simulink model "nmpc_sim"  (R2022a)
settings: Solver=ode4  StartTime=0.0  StopTime=30  FixedStep=0.0005  RelTol=1e-3
model workspace (MAT data in the model file):
  deg2rad = 0.0174532925199
  g2ms2 = 9.81
  kph2ms = 0.277777777778
  rad2deg = 57.2957795131
  rpm2rads = 0.10471975512
values from neighbouring files (symbols this model uses):
  N = 30    [plot_sim_results.m]
  Ts = T/N    (= 0.05)    [plot_sim_results.m]
undefined symbols (not defined in the file or in its folder): index_max, kappar, lbx_0, n_s, np, nu, nx, param_traj_0, phir, s_star_0, sr, u_s, ubx_0, V_star_0, veh, vr, wl, wr, x0, x_s, xr, yr
libraries: simulink x1
settings Model: Creator=Ting  LastModifiedBy=Ting
settings SolverCC: AlgebraicLoopSolver=TrustRegion
settings DebuggingCC: ArithmeticOperatorsInVariantConditions=warning
settings SFSimCC: CustomCodeUndefinedFunction=UseInterfaceOnly
settings CodeAppCC: StateflowObjectComments=on

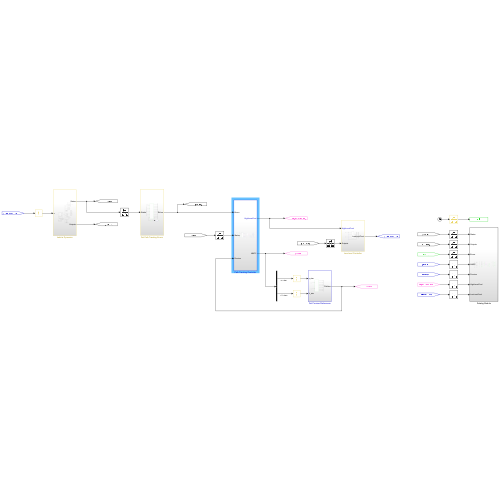
[thumbnail: Simulink's stored preview of the top-level diagram]
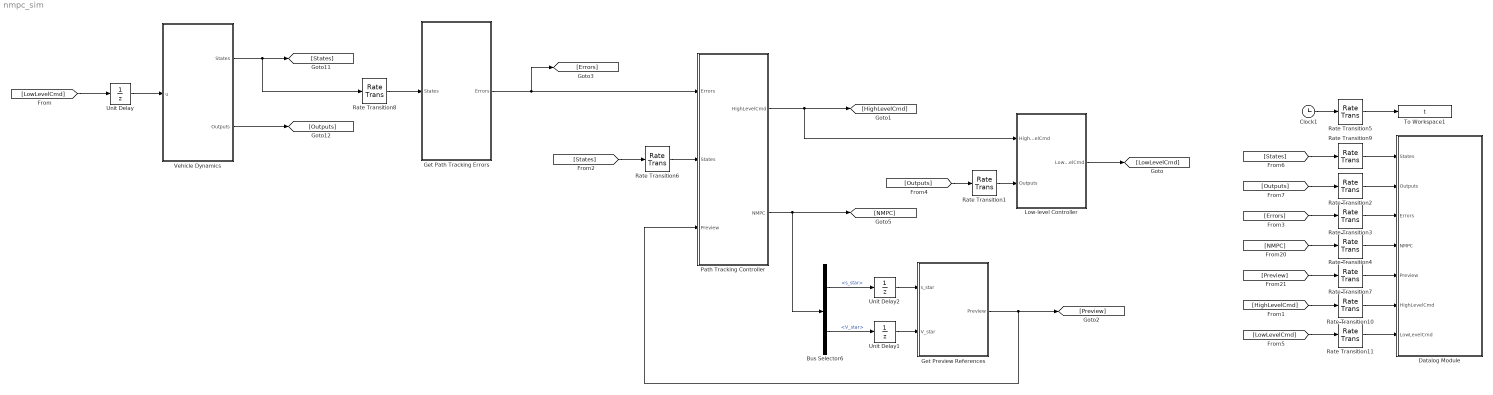
== system nmpc_sim ==
  Bus Selector6 : BusSelector  OutputSignals=s_star,V_star
  Clock1 : Clock
  Datalog Module : Subsystem
  "Get Path Tracking Errors " : Subsystem
  Get Preview References : Subsystem
  Low-level Controller : Subsystem
  Path Tracking Controller : Subsystem
  Rate Transition1 : RateTransition  OutPortSampleTime=Ts
  Rate Transition{2..5,7,9..11} (8 alike) : RateTransition  OutPortSampleTime=Ts_log
  Rate Transition6 : RateTransition  OutPortSampleTime=Ts
  Rate Transition8 : RateTransition  OutPortSampleTime=Ts
  To Workspace1 : ToWorkspace  VariableName=t  SampleTime=-1
      settings: Save2DSignal=2-D array (concatenate along first dimension)
  Unit Delay : UnitDelay  InitialCondition=zeros(7,1)  SampleTime=-1  HasFrameUpgradeWarning=on
  Unit Delay1 : UnitDelay  InitialCondition=V_star_0  SampleTime=-1  HasFrameUpgradeWarning=on
  Unit Delay2 : UnitDelay  InitialCondition=s_star_0  SampleTime=-1  HasFrameUpgradeWarning=on
  Vehicle Dynamics : Subsystem
  wires:
  Rate Transition5/1 -> To Workspace1/1
  Clock1/1 -> Rate Transition5/1
  [States] -> Rate Transition6/1
  Low-level Controller/1(LowLevelCmd) -> [LowLevelCmd]
  Path Tracking Controller/1(HighLevelCmd) -> Low-level Controller/1(HighLevelCmd), [HighLevelCmd]
  [Outputs] -> Rate Transition2/1
  [Outputs] -> Rate Transition1/1
  Unit Delay/1 -> Vehicle Dynamics/1(u)
  [Errors] -> Rate Transition3/1
  Get Preview References/1(Preview) -> Path Tracking Controller/3(Preview), [Preview]
  Rate Transition6/1 -> Path Tracking Controller/2(States)
  "Get Path Tracking Errors "/1(Errors) -> Path Tracking Controller/1(Errors), [Errors]
  Rate Transition8/1 -> "Get Path Tracking Errors "/1(States)
  Path Tracking Controller/2(NMPC) -> [NMPC], Bus Selector6/1
  Bus Selector6/2 -> Unit Delay1/1  "<V_star>"
  Bus Selector6/1 -> Unit Delay2/1  "<s_star>"
  [LowLevelCmd] -> Unit Delay/1
  Vehicle Dynamics/1(States) -> [States], Rate Transition8/1
  Vehicle Dynamics/2(Outputs) -> [Outputs]
  Unit Delay2/1 -> Get Preview References/1(s_star)
  Unit Delay1/1 -> Get Preview References/2(V_star)
  [States] -> Rate Transition9/1
  [HighLevelCmd] -> Rate Transition10/1
  [LowLevelCmd] -> Rate Transition11/1
  [NMPC] -> Rate Transition4/1
  [Preview] -> Rate Transition7/1
  Rate Transition9/1 -> Datalog Module/1(States)
  Rate Transition2/1 -> Datalog Module/2(Outputs)
  Rate Transition3/1 -> Datalog Module/3(Errors)
  Rate Transition4/1 -> Datalog Module/4(NMPC)
  Rate Transition7/1 -> Datalog Module/5(Preview)
  Rate Transition10/1 -> Datalog Module/6(HighLevelCmd)
  Rate Transition11/1 -> Datalog Module/7(LowLevelCmd)
  Rate Transition1/1 -> Low-level Controller/2(Outputs)

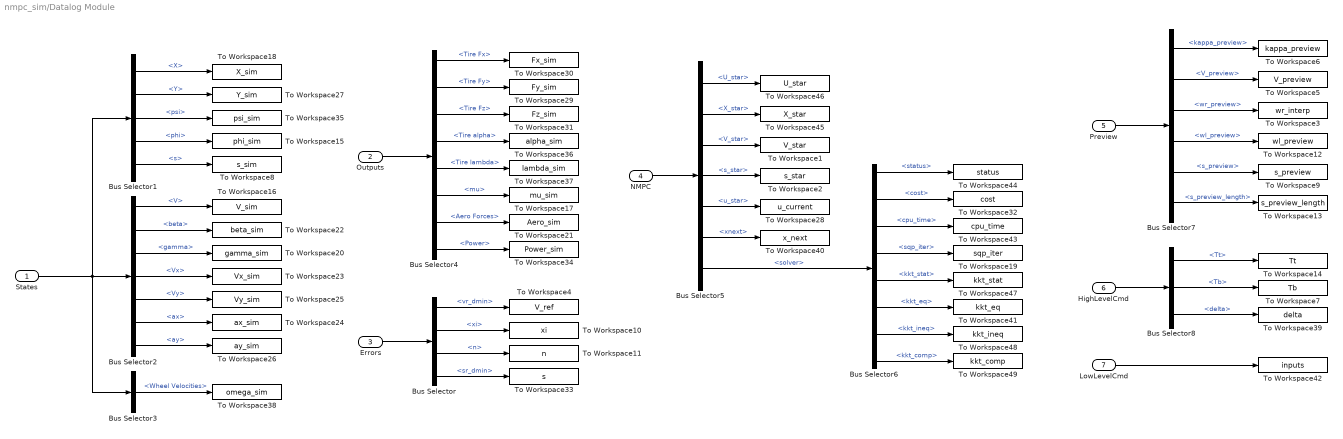
== system nmpc_sim/Datalog Module ==
  States : Inport
  Outputs : Inport  Port=2
  Errors : Inport  Port=3
  NMPC : Inport  Port=4
  Preview : Inport  Port=5
  HighLevelCmd : Inport  Port=6
  LowLevelCmd : Inport  Port=7
  Bus Selector : BusSelector  OutputSignals=vr_dmin,xi,n,sr_dmin
  Bus Selector1 : BusSelector  OutputSignals=Pose.X,Pose.Y,Pose.psi,Pose.phi,Pose.s
  Bus Selector2 : BusSelector  OutputSignals=Motion.V,Motion.beta,Motion.gamma,Motion.Vx,Motion.Vy,Motion.ax,Motion.ay
  Bus Selector3 : BusSelector  OutputSignals=Wheel Velocities
  Bus Selector4 : BusSelector  OutputSignals=Tire Fx,Tire Fy,Tire Fz,Tire alpha,Tire lambda,mu,Aero Forces,Power
  Bus Selector5 : BusSelector  OutputSignals=U_star,X_star,V_star,s_star,u_star,xnext,solver
  Bus Selector6 : BusSelector  OutputSignals=status,cost,cpu_time,sqp_iter,kkt_stat,kkt_eq,kkt_ineq,kkt_comp
  Bus Selector7 : BusSelector  OutputSignals=kappa_preview,V_preview,wr_preview,wl_preview,s_preview,s_preview_length
  Bus Selector8 : BusSelector  OutputSignals=Tt,Tb,delta
  To Workspace1 : ToWorkspace  VariableName=V_star  SampleTime=-1
  To Workspace10 : ToWorkspace  VariableName=xi  SampleTime=-1
  To Workspace11 : ToWorkspace  VariableName=n  SampleTime=-1
  To Workspace12 : ToWorkspace  VariableName=wl_preview  SampleTime=-1
  To Workspace13 : ToWorkspace  VariableName=s_preview_length  SampleTime=0.01
  To Workspace14 : ToWorkspace  VariableName=Tt  SampleTime=-1
      settings: Save2DSignal=2-D array (concatenate along first dimension)
  To Workspace15 : ToWorkspace  VariableName=phi_sim  SampleTime=-1
      settings: Save2DSignal=2-D array (concatenate along first dimension)
  To Workspace16 : ToWorkspace  VariableName=V_sim  SampleTime=-1
      settings: Save2DSignal=2-D array (concatenate along first dimension)
  To Workspace17 : ToWorkspace  VariableName=mu_sim  SampleTime=-1
  To Workspace18 : ToWorkspace  VariableName=X_sim  SampleTime=-1
      settings: Save2DSignal=2-D array (concatenate along first dimension)
  To Workspace19 : ToWorkspace  VariableName=sqp_iter  SampleTime=-1
      settings: Save2DSignal=2-D array (concatenate along first dimension)
  To Workspace2 : ToWorkspace  VariableName=s_star  SampleTime=-1
  To Workspace20 : ToWorkspace  VariableName=gamma_sim  SampleTime=-1
      settings: Save2DSignal=2-D array (concatenate along first dimension)
  To Workspace21 : ToWorkspace  VariableName=Aero_sim  SampleTime=-1
  To Workspace22 : ToWorkspace  VariableName=beta_sim  SampleTime=-1
      settings: Save2DSignal=2-D array (concatenate along first dimension)
  To Workspace23 : ToWorkspace  VariableName=Vx_sim  SampleTime=-1
      settings: Save2DSignal=2-D array (concatenate along first dimension)
  To Workspace24 : ToWorkspace  VariableName=ax_sim  SampleTime=-1
      settings: Save2DSignal=2-D array (concatenate along first dimension)
  To Workspace25 : ToWorkspace  VariableName=Vy_sim  SampleTime=-1
      settings: Save2DSignal=2-D array (concatenate along first dimension)
  To Workspace26 : ToWorkspace  VariableName=ay_sim  SampleTime=-1
      settings: Save2DSignal=2-D array (concatenate along first dimension)
  To Workspace27 : ToWorkspace  VariableName=Y_sim  SampleTime=-1
      settings: Save2DSignal=2-D array (concatenate along first dimension)
  To Workspace28 : ToWorkspace  VariableName=u_current  SampleTime=-1
      settings: Save2DSignal=2-D array (concatenate along first dimension)
  To Workspace29 : ToWorkspace  VariableName=Fy_sim  SampleTime=-1
  To Workspace3 : ToWorkspace  VariableName=wr_interp  SampleTime=-1
  To Workspace30 : ToWorkspace  VariableName=Fx_sim  SampleTime=-1
  To Workspace31 : ToWorkspace  VariableName=Fz_sim  SampleTime=-1
  To Workspace32 : ToWorkspace  VariableName=cost  SampleTime=-1
      settings: Save2DSignal=2-D array (concatenate along first dimension)
  To Workspace33 : ToWorkspace  VariableName=s  SampleTime=-1
  To Workspace34 : ToWorkspace  VariableName=Power_sim  SampleTime=-1
  To Workspace35 : ToWorkspace  VariableName=psi_sim  SampleTime=-1
      settings: Save2DSignal=2-D array (concatenate along first dimension)
  To Workspace36 : ToWorkspace  VariableName=alpha_sim  SampleTime=-1
  To Workspace37 : ToWorkspace  VariableName=lambda_sim  SampleTime=-1
  To Workspace38 : ToWorkspace  VariableName=omega_sim  SampleTime=-1
  To Workspace39 : ToWorkspace  VariableName=delta  SampleTime=-1
      settings: Save2DSignal=2-D array (concatenate along first dimension)
  To Workspace4 : ToWorkspace  VariableName=V_ref  SampleTime=-1
  To Workspace40 : ToWorkspace  VariableName=x_next  SampleTime=-1
      settings: Save2DSignal=2-D array (concatenate along first dimension)
  To Workspace41 : ToWorkspace  VariableName=kkt_eq  SampleTime=-1
      settings: Save2DSignal=2-D array (concatenate along first dimension)
  To Workspace42 : ToWorkspace  VariableName=inputs  SampleTime=-1
      settings: Save2DSignal=2-D array (concatenate along first dimension)
  To Workspace43 : ToWorkspace  VariableName=cpu_time  SampleTime=-1
      settings: Save2DSignal=2-D array (concatenate along first dimension)
  To Workspace44 : ToWorkspace  VariableName=status  SampleTime=-1
      settings: Save2DSignal=2-D array (concatenate along first dimension)
  To Workspace45 : ToWorkspace  VariableName=X_star  SampleTime=-1
  To Workspace46 : ToWorkspace  VariableName=U_star  SampleTime=-1
  To Workspace47 : ToWorkspace  VariableName=kkt_stat  SampleTime=-1
      settings: Save2DSignal=2-D array (concatenate along first dimension)
  To Workspace48 : ToWorkspace  VariableName=kkt_ineq  SampleTime=-1
      settings: Save2DSignal=2-D array (concatenate along first dimension)
  To Workspace49 : ToWorkspace  VariableName=kkt_comp  SampleTime=-1
      settings: Save2DSignal=2-D array (concatenate along first dimension)
  To Workspace5 : ToWorkspace  VariableName=V_preview  SampleTime=-1
  To Workspace6 : ToWorkspace  VariableName=kappa_preview  SampleTime=-1
  To Workspace7 : ToWorkspace  VariableName=Tb  SampleTime=-1
      settings: Save2DSignal=2-D array (concatenate along first dimension)
  To Workspace8 : ToWorkspace  VariableName=s_sim  SampleTime=-1
      settings: Save2DSignal=2-D array (concatenate along first dimension)
  To Workspace9 : ToWorkspace  VariableName=s_preview  SampleTime=-1
  wires:
  States/1 -> Bus Selector1/1, Bus Selector3/1, Bus Selector2/1
  Bus Selector2/5 -> To Workspace25/1  "<Vy>"
  Bus Selector1/2 -> To Workspace27/1  "<Y>"
  Bus Selector1/5 -> To Workspace8/1  "<s>"
  Bus Selector1/1 -> To Workspace18/1  "<X>"
  Bus Selector2/7 -> To Workspace26/1  "<ay>"
  Bus Selector1/3 -> To Workspace35/1  "<psi>"
  Bus Selector2/3 -> To Workspace20/1  "<gamma>"
  Bus Selector2/6 -> To Workspace24/1  "<ax>"
  Bus Selector1/4 -> To Workspace15/1  "<phi>"
  Bus Selector3/1 -> To Workspace38/1  "<Wheel Velocities>"
  Bus Selector2/2 -> To Workspace22/1  "<beta>"
  Bus Selector2/1 -> To Workspace16/1  "<V>"
  Bus Selector2/4 -> To Workspace23/1  "<Vx>"
  Bus Selector4/6 -> To Workspace17/1  "<mu>"
  Bus Selector4/3 -> To Workspace31/1  "<Tire Fz>"
  Bus Selector4/7 -> To Workspace21/1  "<Aero Forces>"
  Outputs/1 -> Bus Selector4/1
  Bus Selector4/5 -> To Workspace37/1  "<Tire lambda>"
  Bus Selector4/1 -> To Workspace30/1  "<Tire Fx>"
  Bus Selector4/4 -> To Workspace36/1  "<Tire alpha>"
  Bus Selector4/2 -> To Workspace29/1  "<Tire Fy>"
  Bus Selector4/8 -> To Workspace34/1  "<Power>"
  Bus Selector/2 -> To Workspace10/1  "<xi>"
  Bus Selector/4 -> To Workspace33/1  "<sr_dmin>"
  Bus Selector/1 -> To Workspace4/1  "<vr_dmin>"
  Bus Selector/3 -> To Workspace11/1  "<n>"
  Errors/1 -> Bus Selector/1
  NMPC/1 -> Bus Selector5/1
  Bus Selector5/1 -> To Workspace46/1  "<U_star>"
  Bus Selector5/2 -> To Workspace45/1  "<X_star>"
  Bus Selector5/3 -> To Workspace1/1  "<V_star>"
  Bus Selector5/4 -> To Workspace2/1  "<s_star>"
  Bus Selector5/5 -> To Workspace28/1  "<u_star>"
  Bus Selector5/6 -> To Workspace40/1  "<xnext>"
  Bus Selector5/7 -> Bus Selector6/1  "<solver>"
  Bus Selector6/1 -> To Workspace44/1  "<status>"
  Bus Selector6/2 -> To Workspace32/1  "<cost>"
  Bus Selector6/3 -> To Workspace43/1  "<cpu_time>"
  Bus Selector6/4 -> To Workspace19/1  "<sqp_iter>"
  Bus Selector6/5 -> To Workspace47/1  "<kkt_stat>"
  Bus Selector6/6 -> To Workspace41/1  "<kkt_eq>"
  Bus Selector6/7 -> To Workspace48/1  "<kkt_ineq>"
  Bus Selector6/8 -> To Workspace49/1  "<kkt_comp>"
  Preview/1 -> Bus Selector7/1
  Bus Selector7/1 -> To Workspace6/1  "<kappa_preview>"
  Bus Selector7/2 -> To Workspace5/1  "<V_preview>"
  Bus Selector7/3 -> To Workspace3/1  "<wr_preview>"
  Bus Selector7/4 -> To Workspace12/1  "<wl_preview>"
  Bus Selector7/5 -> To Workspace9/1  "<s_preview>"
  Bus Selector7/6 -> To Workspace13/1  "<s_preview_length>"
  Bus Selector8/3 -> To Workspace39/1  "<delta>"
  Bus Selector8/1 -> To Workspace14/1  "<Tt>"
  Bus Selector8/2 -> To Workspace7/1  "<Tb>"
  HighLevelCmd/1 -> Bus Selector8/1
  LowLevelCmd/1 -> To Workspace42/1

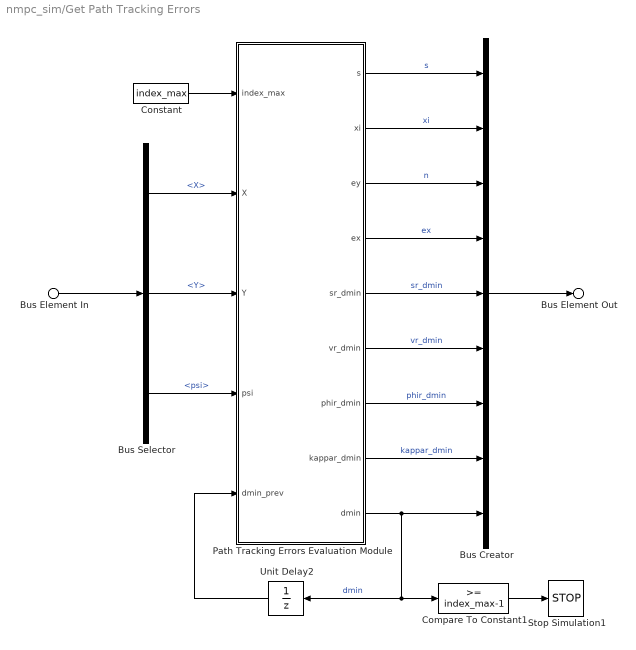
== system nmpc_sim/Get Path Tracking Errors  ==
  Bus Element In : Inport  PortName=States
  Bus Creator : BusCreator  Inputs=9
  Bus Selector : BusSelector  OutputSignals=Pose.X,Pose.Y,Pose.psi
  Compare To Constant1 : simulink/Logic and Bit Operations/Compare To Constant  relop=>=  const=index_max-1  OutDataTypeStr=boolean
  Constant : Constant  Value=index_max
  Path Tracking Errors Evaluation Module : MATLAB Function  TreatAsAtomicUnit=on
  Stop Simulation1 : Stop
  Unit Delay2 : UnitDelay  InitialCondition=1  SampleTime=-1  HasFrameUpgradeWarning=on
  Bus Element Out : Outport  PortName=Errors
  wires:
  Constant/1 -> Path Tracking Errors Evaluation Module/1(index_max)
  Bus Selector/1 -> Path Tracking Errors Evaluation Module/2(X)  "<X>"
  Bus Selector/2 -> Path Tracking Errors Evaluation Module/3(Y)  "<Y>"
  Bus Selector/3 -> Path Tracking Errors Evaluation Module/4(psi)  "<psi>"
  Path Tracking Errors Evaluation Module/9(dmin) -> Bus Creator/9, Unit Delay2/1, Compare To Constant1/1  "dmin"
  Unit Delay2/1 -> Path Tracking Errors Evaluation Module/5(dmin_prev)
  Path Tracking Errors Evaluation Module/2(xi) -> Bus Creator/2  "xi"
  Path Tracking Errors Evaluation Module/3(ey) -> Bus Creator/3  "n"
  Path Tracking Errors Evaluation Module/4(ex) -> Bus Creator/4  "ex"
  Path Tracking Errors Evaluation Module/5(sr_dmin) -> Bus Creator/5  "sr_dmin"
  Path Tracking Errors Evaluation Module/6(vr_dmin) -> Bus Creator/6  "vr_dmin"
  Path Tracking Errors Evaluation Module/7(phir_dmin) -> Bus Creator/7  "phir_dmin"
  Path Tracking Errors Evaluation Module/8(kappar_dmin) -> Bus Creator/8  "kappar_dmin"
  Bus Element In/1 -> Bus Selector/1
  Bus Creator/1 -> Bus Element Out/1
  Compare To Constant1/1 -> Stop Simulation1/1
  Path Tracking Errors Evaluation Module/1(s) -> Bus Creator/1  "s"

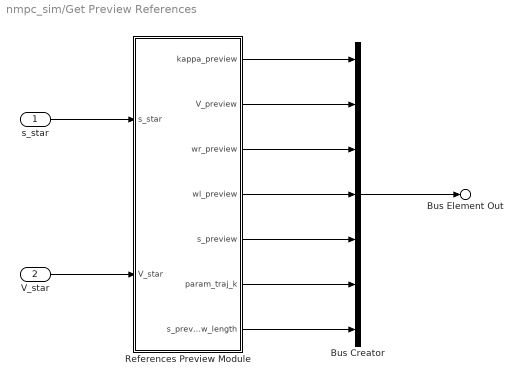
== system nmpc_sim/Get Preview References ==
  s_star : Inport
  V_star : Inport  Port=2
  Bus Creator : BusCreator  Inputs=7
  References Preview Module : MATLAB Function  TreatAsAtomicUnit=on
  Bus Element Out : Outport  PortName=Preview
  wires:
  s_star/1 -> References Preview Module/1(s_star)
  V_star/1 -> References Preview Module/2(V_star)
  References Preview Module/1(kappa_preview) -> Bus Creator/1
  References Preview Module/2(V_preview) -> Bus Creator/2
  References Preview Module/3(wr_preview) -> Bus Creator/3
  References Preview Module/4(wl_preview) -> Bus Creator/4
  References Preview Module/7(s_preview_length) -> Bus Creator/7
  References Preview Module/5(s_preview) -> Bus Creator/5
  References Preview Module/6(param_traj_k) -> Bus Creator/6
  Bus Creator/1 -> Bus Element Out/1

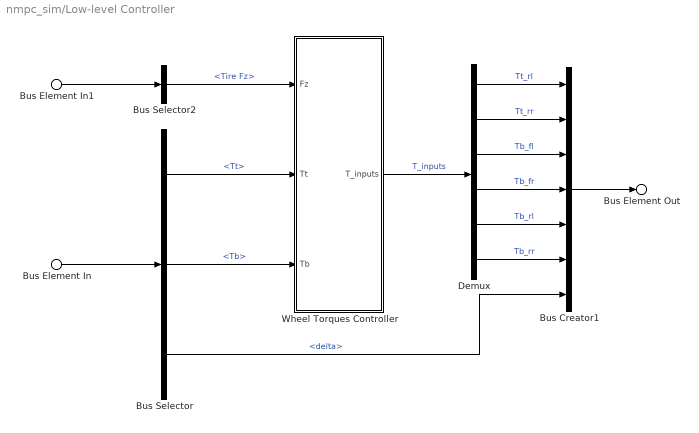
== system nmpc_sim/Low-level Controller ==
  Bus Element In : Inport  PortName=HighLevelCmd
  Bus Element In1 : Inport  Port=2  PortName=Outputs
  Bus Creator1 : BusCreator  Inputs=7
  Bus Selector : BusSelector  OutputSignals=Tt,Tb,delta
  Bus Selector2 : BusSelector  OutputSignals=Tire Fz
  Demux : Demux  Outputs=6
  "Wheel Torques Controller " : MATLAB Function  TreatAsAtomicUnit=on
  Bus Element Out : Outport  PortName=LowLevelCmd
  wires:
  Bus Element In/1 -> Bus Selector/1
  Bus Selector/1 -> "Wheel Torques Controller "/2(Tt)  "<Tt>"
  Bus Selector/2 -> "Wheel Torques Controller "/3(Tb)  "<Tb>"
  "Wheel Torques Controller "/1(T_inputs) -> Demux/1  "T_inputs"
  Bus Element In1/1 -> Bus Selector2/1
  Bus Selector2/1 -> "Wheel Torques Controller "/1(Fz)  "<Tire Fz>"
  Demux/1 -> Bus Creator1/1  "Tt_rl"
  Demux/2 -> Bus Creator1/2  "Tt_rr"
  Demux/3 -> Bus Creator1/3  "Tb_fl"
  Demux/4 -> Bus Creator1/4  "Tb_fr"
  Bus Creator1/1 -> Bus Element Out/1
  Demux/5 -> Bus Creator1/5  "Tb_rl"
  Demux/6 -> Bus Creator1/6  "Tb_rr"
  Bus Selector/3 -> Bus Creator1/7  "<delta>"

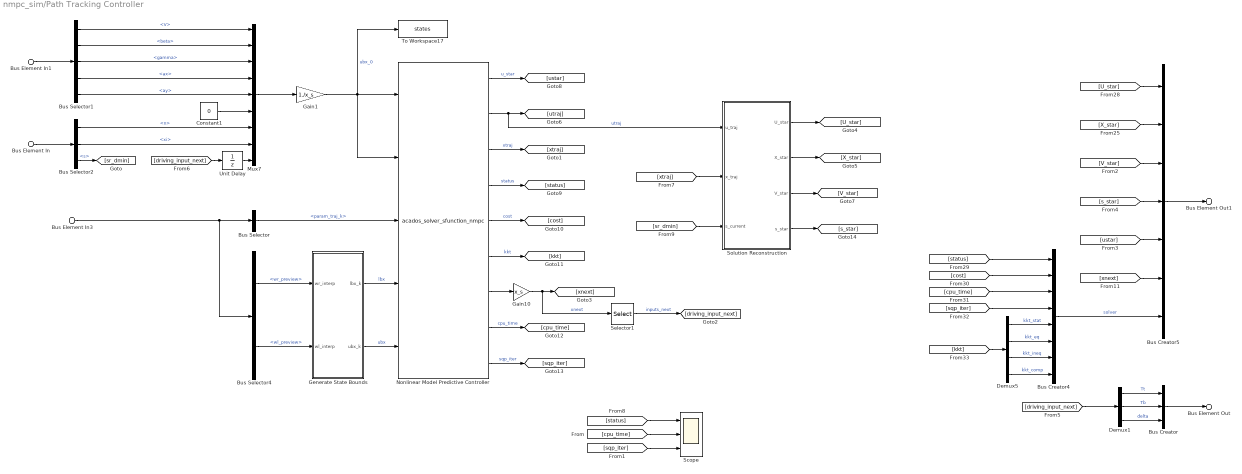
== system nmpc_sim/Path Tracking Controller ==
  Bus Element In : Inport  PortName=Errors
  Bus Element In1 : Inport  Port=2  PortName=States
  Bus Element In3 : Inport  Port=3  PortName=Preview
  Bus Creator : BusCreator  Inputs=3
  Bus Creator4 : BusCreator  Inputs=8
  Bus Creator5 : BusCreator  Inputs=7
  Bus Selector : BusSelector  OutputSignals=param_traj_k
  Bus Selector1 : BusSelector  OutputSignals=Motion.V,Motion.beta,Motion.gamma,Motion.ax,Motion.ay
  Bus Selector2 : BusSelector  OutputSignals=n,xi,s
  Bus Selector4 : BusSelector  OutputSignals=wr_preview,wl_preview
  Constant1 : Constant  Value=0
  Demux1 : Demux  Outputs=3
  Demux5 : Demux
  Gain1 : Gain  Gain=1./x_s
  Gain10 : Gain  Gain=x_s
  Generate State Bounds : MATLAB Function  TreatAsAtomicUnit=on
  Mux7 : Mux  Inputs=[1 1 1 1 1 1 1 1 3]
  Nonlinear Model Predictive Controller : S-Function  FunctionName=acados_solver_sfunction_nmpc  SFunctionDeploymentMode=off  EnableBusSupport=off
      mask Display:
      | global sfun_input_names sfun_output_names
      | for i = 1:length(sfun_input_names)
      | 	port_label('input', i, sfun_input_names{i})
      | end
      | for i = 1:length(sfun_output_names)
      | 	port_label('output', i, sfun_output_names{i})
      | end
  Scope : Scope  NumInputPorts=3
  Selector1 : Selector  InputPortWidth=11  IndexOptions=Index vector (dialog)  Indices=[9 10 11]  OutputSizes=1
  Solution Reconstruction : MATLAB Function  TreatAsAtomicUnit=on
  To Workspace17 : ToWorkspace  VariableName=states  SampleTime=-1
      settings: Save2DSignal=2-D array (concatenate along first dimension)
  Unit Delay : UnitDelay  InitialCondition=[0 0 0]'  SampleTime=-1  HasFrameUpgradeWarning=on
  Bus Element Out : Outport  PortName=HighLevelCmd
  Bus Element Out1 : Outport  Port=2  PortName=NMPC
  wires:
  Nonlinear Model Predictive Controller/1 -> [ustar]  "u_star"
  Bus Selector1/2 -> Mux7/2  "<beta>"
  Bus Selector2/2 -> Mux7/8  "<xi>"
  Nonlinear Model Predictive Controller/9 -> [sqp_iter]  "sqp_iter"
  Gain1/1 -> Nonlinear Model Predictive Controller/1, Nonlinear Model Predictive Controller/2, To Workspace17/1  "ubx_0"
  Nonlinear Model Predictive Controller/8 -> [cpu_time]  "cpu_time"
  Bus Selector2/1 -> Mux7/7  "<n>"
  Mux7/1 -> Gain1/1
  Bus Selector1/1 -> Mux7/1  "<V>"
  Nonlinear Model Predictive Controller/7 -> Gain10/1
  Nonlinear Model Predictive Controller/2 -> Solution Reconstruction/1(u_traj), [utraj]  "utraj"
  Nonlinear Model Predictive Controller/3 -> [xtraj]  "xtraj"
  Nonlinear Model Predictive Controller/4 -> [status]  "status"
  Generate State Bounds/1(lbx_k) -> Nonlinear Model Predictive Controller/4  "lbx"
  Generate State Bounds/2(ubx_k) -> Nonlinear Model Predictive Controller/5  "ubx"
  Bus Element In1/1 -> Bus Selector1/1
  Bus Element In/1 -> Bus Selector2/1
  Unit Delay/1 -> Mux7/9
  [driving_input_next] -> Unit Delay/1
  Bus Selector1/3 -> Mux7/3  "<gamma>"
  Bus Selector1/4 -> Mux7/4  "<ax>"
  [xtraj] -> Solution Reconstruction/2(x_traj)
  Solution Reconstruction/3(V_star) -> [V_star]
  Solution Reconstruction/4(s_star) -> [s_star]
  Bus Selector1/5 -> Mux7/5  "<ay>"
  Bus Element In3/1 -> Bus Selector/1, Bus Selector4/1
  Bus Selector/1 -> Nonlinear Model Predictive Controller/3  "<param_traj_k>"
  Bus Selector4/1 -> Generate State Bounds/1(wr_interp)  "<wr_preview>"
  Bus Selector4/2 -> Generate State Bounds/2(wl_interp)  "<wl_preview>"
  Solution Reconstruction/1(U_star) -> [U_star]
  Solution Reconstruction/2(X_star) -> [X_star]
  Nonlinear Model Predictive Controller/6 -> [kkt]  "kkt"
  Nonlinear Model Predictive Controller/5 -> [cost]  "cost"
  Demux5/4 -> Bus Creator4/8  "kkt_comp"
  Demux5/3 -> Bus Creator4/7  "kkt_ineq"
  Demux5/1 -> Bus Creator4/5  "kkt_stat"
  Demux5/2 -> Bus Creator4/6  "kkt_eq"
  Gain10/1 -> Selector1/1, [xnext]  "xnext"
  [ustar] -> Bus Creator5/5
  [U_star] -> Bus Creator5/1
  [X_star] -> Bus Creator5/2
  [xnext] -> Bus Creator5/6
  [status] -> Bus Creator4/1
  [cost] -> Bus Creator4/2
  [kkt] -> Demux5/1
  [cpu_time] -> Bus Creator4/3
  [sqp_iter] -> Bus Creator4/4
  Bus Creator4/1 -> Bus Creator5/7  "solver"
  Bus Creator5/1 -> Bus Element Out1/1
  [V_star] -> Bus Creator5/3
  [s_star] -> Bus Creator5/4
  Selector1/1 -> [driving_input_next]  "inputs_next"
  Demux1/2 -> Bus Creator/2  "Tb"
  Bus Creator/1 -> Bus Element Out/1
  Demux1/3 -> Bus Creator/3  "delta"
  Demux1/1 -> Bus Creator/1  "Tt"
  [driving_input_next] -> Demux1/1
  [cpu_time] -> Scope/2
  [sqp_iter] -> Scope/3
  Constant1/1 -> Mux7/6
  [sr_dmin] -> Solution Reconstruction/3(s_current)
  Bus Selector2/3 -> [sr_dmin]  "<s>"
  [status] -> Scope/1

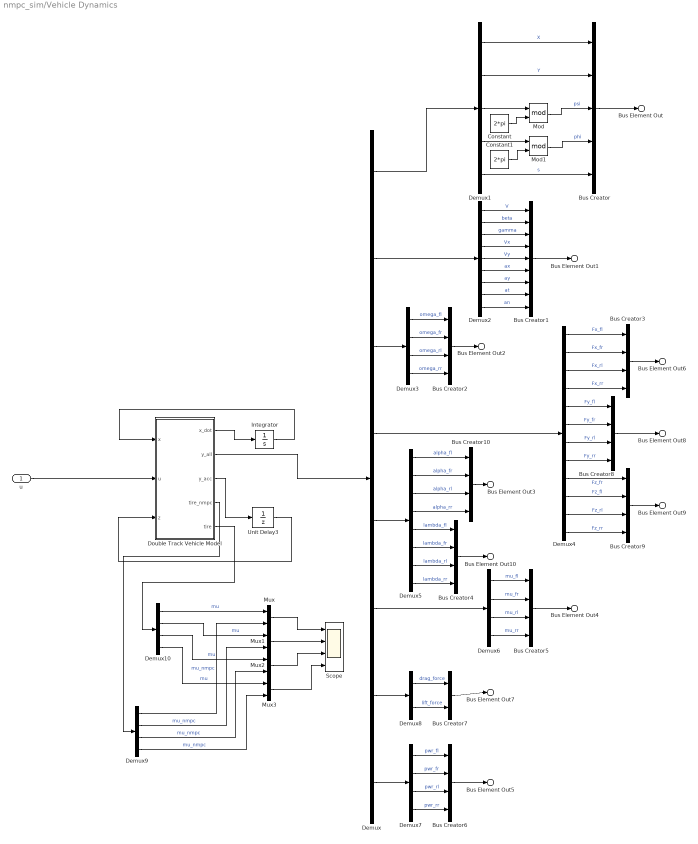
== system nmpc_sim/Vehicle Dynamics ==
  u : Inport
  Bus Creator : BusCreator  Inputs=5
  Bus Creator1 : BusCreator  Inputs=9
  Bus Creator{2..6,8..10} (8 alike) : BusCreator  Inputs=4
  Bus Creator7 : BusCreator  Inputs=2
  Constant : Constant  Value=2*pi
  Constant1 : Constant  Value=2*pi
  Demux : Demux  Outputs=[5 9 4 12 8 4 2 4]
  Demux1 : Demux  Outputs=5
  Demux{3,6..7,9..10} (5 alike) : Demux
  Demux2 : Demux  Outputs=9
  Demux4 : Demux  Outputs=12
  Demux5 : Demux  Outputs=8
  Demux8 : Demux  Outputs=2
  Double Track Vehicle Model : MATLAB Function  TreatAsAtomicUnit=on
  Integrator : Integrator  InitialCondition=x0
  Mod : Math  Operator=mod  SignedPower=on
  Mod1 : Math  Operator=mod  SignedPower=on
  Mux{,1..3} (4 alike) : Mux  Inputs=2
  Scope : Scope  NumInputPorts=4
  Unit Delay3 : UnitDelay  InitialCondition=[0; 0];  SampleTime=-1  HasFrameUpgradeWarning=on
  Bus Element Out : Outport  PortName=States  Element=Pose
  Bus Element Out2 : Outport  PortName=States  Element=Wheel Velocities
  Bus Element Out1 : Outport  PortName=States  Element=Motion
  Bus Element Out3 : Outport  Port=2  PortName=Outputs  Element=Tire alpha
  Bus Element Out4 : Outport  Port=2  PortName=Outputs  Element=mu
  Bus Element Out5 : Outport  Port=2  PortName=Outputs  Element=Power
  Bus Element Out7 : Outport  Port=2  PortName=Outputs  Element=Aero Forces
  Bus Element Out8 : Outport  Port=2  PortName=Outputs  Element=Tire Fy
  Bus Element Out6 : Outport  Port=2  PortName=Outputs  Element=Tire Fx
  Bus Element Out9 : Outport  Port=2  PortName=Outputs  Element=Tire Fz
  Bus Element Out10 : Outport  Port=2  PortName=Outputs  Element=Tire lambda
  wires:
  Double Track Vehicle Model/3(y_acc) -> Unit Delay3/1
  Unit Delay3/1 -> Double Track Vehicle Model/3(z)
  Double Track Vehicle Model/1(x_dot) -> Integrator/1
  Double Track Vehicle Model/2(y_all) -> Demux/1
  u/1 -> Double Track Vehicle Model/2(u)
  Integrator/1 -> Double Track Vehicle Model/1(x)
  Demux1/2 -> Bus Creator/2  "Y"
  Demux1/1 -> Bus Creator/1  "X"
  Demux1/3 -> Mod/1
  Demux1/4 -> Mod1/1
  Bus Creator/1 -> Bus Element Out/1
  Demux/2 -> Demux2/1
  Demux2/1 -> Bus Creator1/1  "V"
  Demux2/2 -> Bus Creator1/2  "beta"
  Demux2/3 -> Bus Creator1/3  "gamma"
  Demux2/4 -> Bus Creator1/4  "Vx"
  Demux2/5 -> Bus Creator1/5  "Vy"
  Demux2/6 -> Bus Creator1/6  "ax"
  Demux2/7 -> Bus Creator1/7  "ay"
  Bus Creator2/1 -> Bus Element Out2/1
  Demux3/4 -> Bus Creator2/4  "omega_rr"
  Demux3/3 -> Bus Creator2/3  "omega_rl"
  Demux3/1 -> Bus Creator2/1  "omega_fl"
  Demux3/2 -> Bus Creator2/2  "omega_fr"
  Demux/3 -> Demux3/1
  Demux/4 -> Demux4/1
  Demux4/1 -> Bus Creator3/1  "Fx_fl"
  Demux4/2 -> Bus Creator3/2  "Fx_fr"
  Demux4/3 -> Bus Creator3/3  "Fx_rl"
  Demux4/4 -> Bus Creator3/4  "Fx_rr"
  Demux4/5 -> Bus Creator8/1  "Fy_fl"
  Demux4/6 -> Bus Creator8/2  "Fy_fr"
  Demux4/7 -> Bus Creator8/3  "Fy_rl"
  Demux4/8 -> Bus Creator8/4  "Fy_rr"
  Demux4/9 -> Bus Creator9/1  "Fz_fr"
  Demux4/10 -> Bus Creator9/2  "Fz_fl"
  Demux4/11 -> Bus Creator9/3  "Fz_rl"
  Demux4/12 -> Bus Creator9/4  "Fz_rr"
  Bus Creator3/1 -> Bus Element Out6/1
  Bus Creator1/1 -> Bus Element Out1/1
  Demux/5 -> Demux5/1
  Demux5/1 -> Bus Creator10/1  "alpha_fl"
  Demux5/2 -> Bus Creator10/2  "alpha_fr"
  Demux5/3 -> Bus Creator10/3  "alpha_rl"
  Demux5/4 -> Bus Creator10/4  "alpha_rr"
  Demux5/5 -> Bus Creator4/1  "lambda_fl"
  Demux5/6 -> Bus Creator4/2  "lambda_fr"
  Demux5/7 -> Bus Creator4/3  "lambda_rl"
  Demux5/8 -> Bus Creator4/4  "lambda_rr"
  Bus Creator10/1 -> Bus Element Out3/1
  Demux/6 -> Demux6/1
  Demux6/2 -> Bus Creator5/2  "mu_fr"
  Demux6/3 -> Bus Creator5/3  "mu_rl"
  Demux6/4 -> Bus Creator5/4  "mu_rr"
  Bus Creator5/1 -> Bus Element Out4/1
  Demux6/1 -> Bus Creator5/1  "mu_fl"
  Bus Creator6/1 -> Bus Element Out5/1
  Demux7/4 -> Bus Creator6/4  "pwr_rr"
  Demux7/3 -> Bus Creator6/3  "pwr_rl"
  Demux7/2 -> Bus Creator6/2  "pwr_fr"
  Demux/8 -> Demux7/1
  Demux7/1 -> Bus Creator6/1  "pwr_fl"
  Demux/7 -> Demux8/1
  Demux8/1 -> Bus Creator7/1  "drag_force"
  Demux8/2 -> Bus Creator7/2  "lift_force"
  Bus Creator7/1 -> Bus Element Out7/1
  Demux1/5 -> Bus Creator/5  "s"
  Bus Creator8/1 -> Bus Element Out8/1
  Bus Creator9/1 -> Bus Element Out9/1
  Bus Creator4/1 -> Bus Element Out10/1
  Mod/1 -> Bus Creator/3  "psi"
  Constant/1 -> Mod/2
  Mod1/1 -> Bus Creator/4  "phi"
  Constant1/1 -> Mod1/2
  Demux/1 -> Demux1/1
  Double Track Vehicle Model/4(tire_nmpc) -> Demux9/1
  Demux9/1 -> Mux/2  "mu_nmpc"
  Demux9/2 -> Mux1/2  "mu_nmpc"
  Demux9/3 -> Mux2/2  "mu_nmpc"
  Demux9/4 -> Mux3/2  "mu_nmpc"
  Double Track Vehicle Model/5(tire) -> Demux10/1
  Demux10/1 -> Mux/1  "mu"
  Demux10/2 -> Mux1/1  "mu"
  Demux10/3 -> Mux2/1  "mu"
  Demux10/4 -> Mux3/1  "mu"
  Mux/1 -> Scope/1
  Mux1/1 -> Scope/2
  Mux2/1 -> Scope/3
  Mux3/1 -> Scope/4
  Demux2/8 -> Bus Creator1/8  "at"
  Demux2/9 -> Bus Creator1/9  "an"

== matlab function nmpc_sim/Get Preview References/References Preview Module ==
  data: s_star input; V_star input; param_traj_0 parameter; np parameter; sr parameter; vr parameter; kappar parameter; kappa_preview output; V_preview output; wr_preview output; wl_preview output; s_preview output; param_traj_k output; s_preview_length output; wr parameter; wl parameter; Ts parameter
function [kappa_preview, V_preview, wr_preview, wl_preview, s_preview , param_traj_k, s_preview_length] = fcn(s_star, V_star, param_traj_0, np, sr, vr, kappar, wr, wl, Ts)

s_preview = [s_star(2:end); s_star(end)+V_star(end)*Ts];

kappa_preview = interp1(sr,kappar,s_preview,"linear",'extrap');
V_preview = interp1(sr,vr,s_preview,"linear",'extrap');
wr_preview = interp1(sr,wr,s_preview,"linear",'extrap');
wl_preview = interp1(sr,wl,s_preview,"linear",'extrap');

param_traj_0(1:np:end) = kappa_preview;
param_traj_0(2:np:end) = V_preview;

param_traj_k = param_traj_0;

s_preview_length = s_preview(end)-s_star(1);


end

== matlab function nmpc_sim/Path Tracking Controller/Solution Reconstruction ==
  data: u_traj input; x_traj input; s_current input; U_star output; X_star output; V_star output; s_star output; nu parameter; nx parameter; N parameter; u_s parameter; x_s parameter
function [U_star,X_star,V_star,s_star] = fcn(u_traj, x_traj, s_current, nu, nx, N,u_s, x_s)

U_star = reshape(u_traj,nu,N)'.*u_s';
X_star = reshape(x_traj,nx,N+1)'.*x_s';


V_star = X_star(:,1);
s_star = X_star(:,6) + s_current;






end

== matlab function nmpc_sim/Vehicle Dynamics/Double Track Vehicle Model ==
  data: x input; u input; z input; x_dot output; y_all output; veh parameter; y_acc output; tire_nmpc output; tire output
function [x_dot,y_all,y_acc,tire_nmpc,tire]  = fcn(x,u,z,veh)
%% States
V = x(1);
beta = x(2);
gamma = x(3);
omega_fl = x(4);
omega_fr = x(5);
omega_rl = x(6);
omega_rr = x(7);

X = x(8);
Y = x(9);
phi = x(10);
s = x(11);

psi = phi - beta;


%% Aux. variables
ax_bar = z(1);
ay_bar = z(2);


%% Inputs
% Wheel torque
Tt_rl = u(1);
Tt_rr = u(2);
Tb_fl = u(3);
Tb_fr = u(4);
Tb_rl = u(5);
Tb_rr = u(6);
delta = u(7);
% Tfl = u(1);
% Tfr = u(2);
% Trl = u(3);
% Trr = u(4);
% delta = u(5);


%% Vehicle model - equations
%Calculate variables of the system other than the states and inputs

cosd = cos(delta);
sind = sin(delta);
cosb = cos(beta);
sinb = sin(beta);
cosbd = cos(beta-delta);
sinbd = sin(beta-delta);


% longitudinal and lateral velocities
vx = V*cosb;
vy = V*sinb;

% Resistance forces
%-aerodynamic forces [N]
f_drag = 0.5*veh.drag_coeff*vx^2;
f_lift = 0.5*veh.lift_coeff*vx^2;


% Tire velocities

vxfl = (vx-0.5*veh.wt*gamma)*cosd + (vy+veh.lf*gamma)*sind;
vxfr = (vx+0.5*veh.wt*gamma)*cosd + (vy+veh.lf*gamma)*sind;
vxrl = (vx-0.5*veh.wt*gamma);
vxrr = (vx+0.5*veh.wt*gamma);

vyfl = (vy+veh.lf*gamma)*cosd - (vx-0.5*veh.wt*gamma)*sind;
vyfr = (vy+veh.lf*gamma)*cosd - (vx+0.5*veh.wt*gamma)*sind;
vyrl = (vy-veh.lr*gamma);
vyrr = (vy-veh.lr*gamma);

% Tire sideslip angles
alphafl = atan(vyfl/vxfl);
alphafr = atan(vyfr/vxfr);
alpharl = atan(vyrl/vxrl);
alpharr = atan(vyrr/vxrr);

% Tire longitudinal slips
lambdafl = (veh.rw*omega_fl-vxfl)/vxfl;
lambdafr = (veh.rw*omega_fr-vxfr)/vxfr;
lambdarl = (veh.rw*omega_rl-vxrl)/vxrl;
lambdarr = (veh.rw*omega_rr-vxrr)/vxrr;


% vertical tyre forces [N]
t1 = veh.g*veh.lr/veh.l - ax_bar*veh.hc/veh.l;
t2 = veh.g*veh.lf/veh.l + ax_bar*veh.hc/veh.l;
t3 = veh.hc*ay_bar/veh.wt/veh.g;

fzfl = 0.5*veh.m*t1 - veh.m*t1*t3 - f_lift/4;
fzfr = 0.5*veh.m*t1 + veh.m*t1*t3 - f_lift/4;
fzrl = 0.5*veh.m*t2 - veh.m*t2*t3 - f_lift/4;
fzrr = 0.5*veh.m*t2 + veh.m*t2*t3 - f_lift/4;

fzf = fzfl + fzfr;
fzr = fzrl + fzrr;


% Tire forces
mu = 1.0;

% Tire longitudinal slips
sxfl = lambdafl;
sxfr = lambdafr;
sxrl = lambdarl;
sxrr = lambdarr;

% Tire lateral slips
syfl = vyfl/vxfl;
syfr = vyfr/vxfr;
syrl = vyrl/vxrl;
syrr = vyrr/vxrr;

rho  = 1e-12;
sfl = (sxfl^2+syfl^2 +rho)^0.5;
sfr = (sxfr^2+syfr^2 +rho)^0.5;
srl = (sxrl^2+syrl^2 +rho)^0.5;
srr = (sxrr^2+syrr^2 +rho)^0.5;

fxfl = (sxfl/sfl)*MF_Fx(veh,sfl,fzfl,mu);
fxfr = (sxfr/sfr)*MF_Fx(veh,sfr,fzfr,mu);
fxrl = (sxrl/srl)*MF_Fx(veh,srl,fzrl,mu);
fxrr = (sxrr/srr)*MF_Fx(veh,srr,fzrr,mu);
fxf = fxfl + fxfr;
fxr = fxrl + fxrr;

fyfl = (syfl/sfl)*MF_Fy(veh,sfl,fzfl,mu);
fyfr = (syfr/sfr)*MF_Fy(veh,sfr,fzfr,mu);
fyrl = (syrl/srl)*MF_Fy(veh,srl,fzrl,mu);
fyrr = (syrr/srr)*MF_Fy(veh,srr,fzrr,mu);
fyf = fyfl + fyfr;
fyr = fyrl + fyrr;


mufl = (fxfl^2+fyfl^2)^(0.5)/fzfl;
mufr = (fxfr^2+fyfr^2)^(0.5)/fzfr;
murl = (fxrl^2+fyrl^2)^(0.5)/fzrl;
murr = (fxrr^2+fyrr^2)^(0.5)/fzrr;

Fxfl_nmpc = (Tb_fl)/veh.rw;
Fxfr_nmpc = (Tb_fr)/veh.rw;
Fxrl_nmpc = (Tt_rl+Tb_rl)/veh.rw;
Fxrr_nmpc = (Tt_rr+Tb_rr)/veh.rw;

Fyfl_nmpc = MF_Fy(veh,alphafl,fzfl,mu);
Fyfr_nmpc = MF_Fy(veh,alphafr,fzfr,mu);
Fyrl_nmpc = MF_Fy(veh,alpharl,fzrl,mu);
Fyrr_nmpc = MF_Fy(veh,alpharr,fzrr,mu);

mufl_nmpc = sqrt(Fxfl_nmpc^2 + Fyfl_nmpc^2)/fzfl;
mufr_nmpc = sqrt(Fxfr_nmpc^2 + Fyfr_nmpc^2)/fzfr;
murl_nmpc = sqrt(Fxrl_nmpc^2 + Fyrl_nmpc^2)/fzrl;
murr_nmpc = sqrt(Fxrr_nmpc^2 + Fyrr_nmpc^2)/fzrr;

tire_nmpc = [mufl_nmpc; mufr_nmpc; murl_nmpc; murr_nmpc];
tire = [mufl; mufr; murl; murr];


%% Vehicle model - state derivatives
% Define derivatives of the state-space model

Fx = fxf*cosd + fxr - fyf*sind - f_drag;
Fy = fyf*cosd + fyr + fxf*sind;
ax = Fx/veh.m;
ay = Fy/veh.m;

Mz = veh.lf*(fyf*cosd+fxf*sind) - veh.lr*fyr + 0.5*veh.wt*((fxfr-fxfl)*cosd+(fyfl-fyfr)*sind) + 0.5*veh.wt*(fxrr-fxrl);

% Ft = fxf*cosbd + fxr*cosb + fyf*sinbd + fyr*sinb - f_drag*cosb;
% Fn = fyf*cosbd + fyr*cosb - fxf*sinbd - fxr*sinb + f_drag*sinb;
at = (fxf*cosbd + fxr*cosb + fyf*sinbd + fyr*sinb - f_drag*cosb)/veh.m;
an = (fyf*cosbd + fyr*cosb - fxf*sinbd - fxr*sinb + f_drag*sinb)/veh.m;


% State derivatives equations
x_dot = [
    at;
    an/V-gamma;
    Mz/veh.Iz;
    (Tb_fl - fxfl*veh.rw)/veh.Iw;
    (Tb_fr - fxfr*veh.rw)/veh.Iw;
    (Tt_rl+Tb_rl - fxrl*veh.rw)/veh.Iw;
    (Tt_rr+Tb_rr - fxrr*veh.rw)/veh.Iw;
    V*cos(phi);
    V*sin(phi);
    an/V;
    V;
    ];


%% Outputs
y_acc = [ax; ay];
y_Fx = [fxfl; fxfr; fxrl; fxrr];
y_Fy = [fyfl; fyfr; fyrl; fyrr];
y_Fz = [fzfl; fzfr; fzrl; fzrr];
y_alpha = [alphafl; alphafr; alpharl; alpharr];
y_lambda = [lambdafl; lambdafr; lambdarl; lambdarr];
y_vel = [vx; vy];

y_mu = [mufl; mufr; murl; murr];
y_aero = [f_drag; f_lift];
y_pwr = [Tb_fl*omega_fl; Tb_fr*omega_fr; (Tt_rl+Tb_rl)*omega_rl; (Tt_rr+Tb_rr)*omega_rr];

y_pose = [X; Y; psi; phi; s];
y_motion = [V; beta; gamma; vx; vy; ax; ay; at; an];
y_wheelvel = [omega_fl; omega_fr; omega_rl; omega_rr];
y_tireforces = [y_Fx; y_Fy; y_Fz];
y_tireslips = [y_alpha; y_lambda];


y_all = [y_pose; y_motion; y_wheelvel; y_tireforces; y_tireslips; y_mu; y_aero; y_pwr];
%[5 7 4 12 8 4 2 4]

%% Tire Model

function Fx = MF_Fx(veh,lambda,Fz,mu)
Fx = mu*(veh.d1x*Fz+veh.d2x)*sin(veh.Cx*atan(veh.Bx*lambda));
end

function Fy = MF_Fy(veh,alpha,Fz,mu)
Fy = -mu*(veh.d1y*Fz+veh.d2y)*sin(veh.Cy*atan(veh.By*alpha));
end



end

== matlab function nmpc_sim/Path Tracking Controller/Generate State Bounds ==
  data: wr_interp input; wl_interp input; lbx_k output; ubx_k output; veh parameter; lbx_0 parameter; ubx_0 parameter; nx parameter; N parameter; n_s parameter
function [lbx_k,ubx_k] = fcn(wr_interp, wl_interp, veh, lbx_0, ubx_0, nx, N, n_s)


lbx_0(7:nx:end) = (-wr_interp(2:N)+veh.wt/2)/n_s;
ubx_0(7:nx:end) = (wl_interp(2:N)-veh.wt/2)/n_s;

lbx_k = lbx_0;
ubx_k = ubx_0;

end

== matlab function nmpc_sim/Get Path Tracking Errors /Path Tracking Errors Evaluation Module ==
  data: s output; index_max input; xi output; X input; Y input; psi input; dmin_prev input; ey output; ex output; sr_dmin output; vr_dmin output; phir_dmin output; kappar_dmin output; dmin output; xr parameter; yr parameter; phir parameter; kappar parameter; vr parameter; sr parameter
function [s,xi,ey,ex,sr_dmin,vr_dmin,phir_dmin,kappar_dmin,dmin] = fcn(index_max,X,Y,psi,dmin_prev,xr, yr, phir, kappar, vr, sr)   


%=========== Determine Search Range ===========%
if dmin_prev > index_max
    dmin_prev = 1;
end

d_start = dmin_prev-20;
if d_start < 1
    d_start = 1;
end

d_end = d_start+100;
if d_end > index_max
    d_end = index_max;
end

dmin_search_range = d_start:d_end;


%=========== Find Matching Point ===========%
dmin_arr = (X-xr(dmin_search_range)).^2+(Y-yr(dmin_search_range)).^2;  % calculate euclidean distances
[~,dmin_search] = min(dmin_arr);   % index of matching point
dmin = dmin_search+d_start-1;


%=========== Error Vector Projection ===========%
tvec = [cos(phir(dmin)); sin(phir(dmin))];
nvec = [-sin(phir(dmin)); cos(phir(dmin))];
evec = [X-xr(dmin); Y-yr(dmin)];
ey = nvec'*evec;
ex = tvec'*evec;


%=========== Calculate Station and Reference Heading ===========%
sr_dmin = sr(dmin);
phir_dmin = phir(dmin);
vr_dmin = vr(dmin);
kappar_dmin = kappar(dmin);
projection_point_phir = phir_dmin+kappar_dmin*ex;

s = sr_dmin;


%=========== Calculate Heading Error ===========%
xi = psi-projection_point_phir;

if xi > pi
    xi = xi-2*pi;
elseif xi < -pi
    xi = xi+2*pi;
end


   
    
end

== matlab function nmpc_sim/Low-level Controller/Wheel Torques Controller  ==
  data: Fz input; T_inputs output; Tt input; Tb input
function T_inputs = fcn(Fz,Tt,Tb)

Fzf = Fz(1)+Fz(2);
Fzr = Fz(3)+Fz(4);
dFzf = 0.5*(Fz(2)-Fz(1));
dFzr = 0.5*(Fz(4)-Fz(3));

kbv = 0.6;
Tf = kbv*Tb;
Tr = Tt + (1-kbv)*Tb;

Tb_fl = 0.5*Tf*(1-dFzf/Fzf);
Tb_fr = 0.5*Tf*(1+dFzf/Fzf);

if Tr>0
    Tt_rl = 0.5*Tr*(1-dFzr/Fzr);
    Tt_rr = 0.5*Tr*(1+dFzr/Fzr);
    Tb_rl = 0;
    Tb_rr = 0;
else
    Tt_rl = 0;
    Tt_rr = 0;
    Tb_rl = 0.5*Tr*(1-dFzr/Fzr);
    Tb_rr = 0.5*Tr*(1+dFzr/Fzr);
end


    
% 
% Tfl = 0.5*Tf*(1-dFzf/Fzf);
% Tfr = 0.5*Tf*(1+dFzf/Fzf);
% Trl = 0.5*Tr*(1-dFzr/Fzr);
% Trr = 0.5*Tr*(1+dFzr/Fzr);

% T_inputs = [Tfl; Tfr; Trl; Trr];
T_inputs = [Tt_rl; Tt_rr; Tb_fl; Tb_fr; Tb_rl; Tb_rr];
